simulink model "GFL_inverter"  (R2025a)
settings: Solver=ode4  StartTime=0.0  StopTime=8.5  FixedStep=1e-6  RelTol=1e-3
values from neighbouring files (symbols this model uses):
  An1 = amp1*funn    [dq_saopin_for_GFL_inverter.m]
  An2 = 0    [dq_saopin_for_GFL_inverter.m]
  An3 = 0    [dq_saopin_for_GFL_inverter.m]
  An4 = 0    [dq_saopin_for_GFL_inverter.m]
  An5 = 0    [dq_saopin_for_GFL_inverter.m]
  Ap1 = amp1*funp    [dq_saopin_for_GFL_inverter.m]
  Ap2 = 0    [dq_saopin_for_GFL_inverter.m]
  Ap3 = 0    [dq_saopin_for_GFL_inverter.m]
  Ap4 = 0    [dq_saopin_for_GFL_inverter.m]
  Ap5 = 0    [dq_saopin_for_GFL_inverter.m]
  hp1 = f    [dq_saopin_for_GFL_inverter.m]
  hp2 = f    [dq_saopin_for_GFL_inverter.m]
  hp3 = f    [dq_saopin_for_GFL_inverter.m]
  hp4 = f    [dq_saopin_for_GFL_inverter.m]
  hp5 = f    [dq_saopin_for_GFL_inverter.m]
  t_inj = 7.5    [dq_saopin_for_GFL_inverter.m]
  Ts = 5e-6    (= 5e-06)    [dq_saopin_for_GFL_inverter.m]
undefined symbols (not defined in the file or in its folder): DiscIntNeverNeededParam, level
libraries: powerlib_extras x37, spsControlledVoltageSourceLib x18, spsThreePhaseVIMeasurementLib x7, slpidlib x4, simulink_extras x4, spsabctodq0Lib x3, spsSeriesRLCBranchLib x2, spsUniversalBridgeLib x2, spsMultimeterLib x2, spsThreePhaseProgrammableVoltageSourceLib x1, spsGroundLib x1, spsIGBTDiodeLib x1
(part 2 of 2)

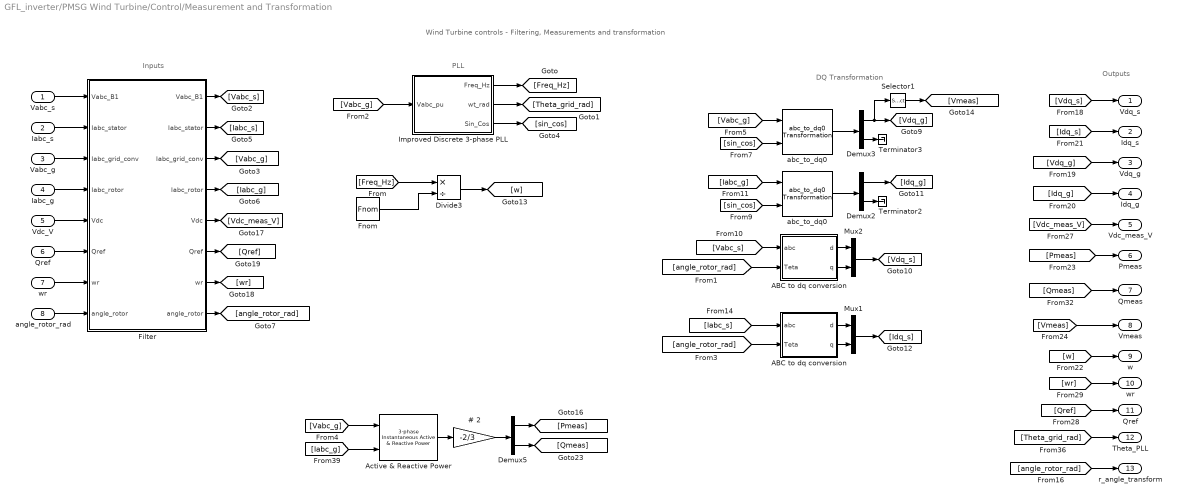
== system GFL_inverter/PMSG Wind Turbine/Control/Measurement and Transformation ==
  note: Wind Turbine controls - Filtering, Measurements and transformation
  note: Outputs
  note: Inputs
  note: PLL
  note: DQ Transformation
  Vabc_s : Inport
  Iabc_s : Inport  Port=2
  Vabc_g : Inport  Port=3
  Iabc_g : Inport  Port=4
  Vdc_V : Inport  Port=5
  Qref : Inport  Port=6
  wr : Inport  Port=7
  angle_rotor_rad : Inport  Port=8
  " Improved Discrete 3-phase PLL" : Subsystem  AncestorBlock=|  mask(Discrete 3-phase PLL){Fmin=0.75*Fnom, Par_Init=[0 Fnom], ParK=[5 3.2 1 50], Ts=Ts}
      | powerlib_extras/Discrete 
      | Control Blocks/Discrete
      | 3-phase PLL
      mask prompts: Fmin "Minimum frequency (Hz):"; Par_Init "Initial inputs:[ Phase(degrees)   Frequency(Hz) ]"; ParK "Regulator gains [ Kp1 Kp2  Ki1  Ki2 ]"; Ts "Sample time:"
      mask help:
      | This Phase Locked Loop (PLL) system can be used  to synchronize on a set of variable frequency, three-phase sinusoidal signals.
      |
      | Input 1: Vector containing the normalized
      |              three-phase signals [Va Vb Vc]
      | Output 1:  Measured frequency (Hz) = w/(2pi)
      | Output 2:  Ramp w.t   varying between  0 and 2*pi,
      | synchronized on zero crossings of the fundamental (positive-sequence) of phase A.
      | Output 3: Vector [sin(wt) cos(wt)]
      mask init:
      | Kp1=ParK(1);
      | Kp2=ParK(2);
      | Ki1=ParK(3);
      | Ki2=ParK(4);
      | Phase_Init=Par_Init(1);
      | Finit=Par_Init(2);
      | power_initmask();
      settings: OpenFcn=power_openblockproxy();
  # 2 : Gain  Gain=-2/3  SaturateOnIntegerOverflow=on  OutDataTypeStr=Inherit: Same as input  ParamDataTypeStr=Inherit: Same as input
  "ABC to dq conversion " : Subsystem
  ABC to dq conversion : Subsystem
  Active & Reactive Power : powerlib_extras/Measurements/3-phase  Instantaneous  Active & Reactive Power
  Demux2 : Demux  Outputs=[2 1]
      settings: DisplayOption=none
  Demux3 : Demux  Outputs=[2 1]
      settings: DisplayOption=none
  Demux5 : Demux  Outputs=2
      settings: DisplayOption=none
  Divide3 : Product  Inputs=*/
  Filter : Subsystem  mask{Freq=1e4, Zeta1=0.707, Ts=Ts}
      mask prompts: Freq "Cut-off frequency (Hz):"; Zeta1 "Damping factor Zeta:"; Ts "Sample time"
  Fnom : Constant  Value=Fnom
  Mux1 : Mux  Inputs=2
  Mux2 : Mux  Inputs=2
  Selector1 : Selector  InputPortWidth=2  IndexOptions=Index vector (dialog)  Indices=1  OutputSizes=[(-2)]
  Terminator2 : Terminator
  Terminator3 : Terminator
  abc_to_dq0 : powerlib_extras/Measurements/abc_to_dq0 Transformation
  "abc_to_dq0 " : powerlib_extras/Measurements/abc_to_dq0 Transformation
  Vdq_s : Outport
  Idq_s : Outport  Port=2
  Vdq_g : Outport  Port=3
  Idq_g : Outport  Port=4
  Vdc_meas_V : Outport  Port=5
  Pmeas : Outport  Port=6
  Qmeas : Outport  Port=7
  Vmeas : Outport  Port=8
  w : Outport  Port=9
  "wr " : Outport  Port=10
  "Qref " : Outport  Port=11
  Theta_PLL : Outport  Port=12
  r_angle_transform : Outport  Port=13
  wires:
  angle_rotor_rad/1 -> Filter/8(angle_rotor)
  Filter/8("angle_rotor ") -> [angle_rotor_rad]
  Filter/7("wr ") -> [wr]
  Filter/6("Qref ") -> [Qref]
  Filter/5("Vdc ") -> [Vdc_meas_V]
  Filter/4("Iabc_rotor ") -> [Iabc_g]
  Filter/3("Iabc_grid_conv ") -> [Vabc_g]
  Filter/2("Iabc_stator ") -> [Iabc_s]
  Filter/1("Vabc_B1 ") -> [Vabc_s]
  [wr] -> "wr "/1
  [Qref] -> "Qref "/1
  [Vdc_meas_V] -> Vdc_meas_V/1
  wr/1 -> Filter/7(wr)
  Qref/1 -> Filter/6(Qref)
  Vdc_V/1 -> Filter/5(Vdc)
  Iabc_g/1 -> Filter/4(Iabc_rotor)
  Vabc_g/1 -> Filter/3(Iabc_grid_conv)
  Iabc_s/1 -> Filter/2(Iabc_stator)
  Vabc_s/1 -> Filter/1(Vabc_B1)
  [angle_rotor_rad] -> "ABC to dq conversion "/2(Teta)
  [Vmeas] -> Vmeas/1
  [Pmeas] -> Pmeas/1
  [w] -> w/1
  [Idq_s] -> Idq_s/1
  [Idq_g] -> Idq_g/1
  [Vdq_g] -> Vdq_g/1
  [Vdq_s] -> Vdq_s/1
  Demux2/1 -> [Idq_g]
  [Iabc_s] -> "ABC to dq conversion "/1(abc)
  [Iabc_g] -> "abc_to_dq0 "/1
  [Vabc_s] -> ABC to dq conversion/1(abc)
  [sin_cos] -> "abc_to_dq0 "/2
  [sin_cos] -> abc_to_dq0/2
  [Vabc_g] -> abc_to_dq0/1
  [Freq_Hz] -> Divide3/1
  Divide3/1 -> [w]
  Fnom/1 -> Divide3/2
  "abc_to_dq0 "/1 -> Demux2/1
  Demux2/2 -> Terminator2/1
  abc_to_dq0/1 -> Demux3/1
  Demux3/2 -> Terminator3/1
  Demux3/1 -> [Vdq_g], Selector1/1
  [Qmeas] -> Qmeas/1
  [Theta_grid_rad] -> Theta_PLL/1
  [angle_rotor_rad] -> r_angle_transform/1
  [Vabc_g] -> " Improved Discrete 3-phase PLL"/1(Vabc_pu)
  " Improved Discrete 3-phase PLL"/2(wt_rad) -> [Theta_grid_rad]
  " Improved Discrete 3-phase PLL"/3(Sin_Cos) -> [sin_cos]
  " Improved Discrete 3-phase PLL"/1(Freq_Hz) -> [Freq_Hz]
  [Vabc_g] -> Active & Reactive Power/1
  [Iabc_g] -> Active & Reactive Power/2
  Demux5/1 -> [Pmeas]
  Demux5/2 -> [Qmeas]
  Active & Reactive Power/1 -> # 2/1
  # 2/1 -> Demux5/1
  Selector1/1 -> [Vmeas]
  [angle_rotor_rad] -> ABC to dq conversion/2(Teta)
  ABC to dq conversion/1(d) -> Mux2/1
  ABC to dq conversion/2(q) -> Mux2/2
  Mux2/1 -> [Vdq_s]
  "ABC to dq conversion "/1(d) -> Mux1/1
  "ABC to dq conversion "/2(q) -> Mux1/2
  Mux1/1 -> [Idq_s]

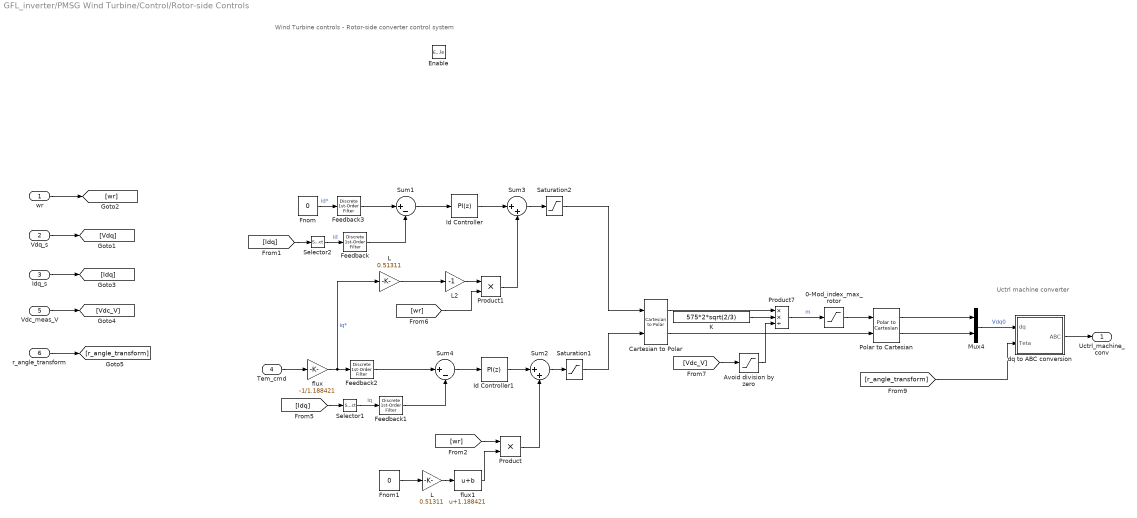
== system GFL_inverter/PMSG Wind Turbine/Control/Rotor-side Controls ==
  note: Wind Turbine controls - Rotor-side converter control system
  note: Uctrl machine converter
  wr : Inport
  " Vdq_s" : Inport  Port=2
  Idq_s : Inport  Port=3
  Tem_cmd : Inport  Port=4
  Vdc_meas_V : Inport  Port=5
  r_angle_transform : Inport  Port=6
  Enable : EnablePort
  0-Mod_index_max_rotor : Saturate  UpperLimit=2  LowerLimit=0
  Avoid division by zero : Saturate  UpperLimit=inf  LowerLimit=1e-6
  Cartesian to Polar : simulink_extras/Transformations/Cartesian to Polar
  Feedback{,1..3} (4 alike) : powerlib_extras/Discrete  Control Blocks/Discrete 1st-Order Filter  FilterType=Lowpass  Tc=Fb_time_const  Ts=Ts  Initialize=on  Vac_Init=[0 -25 60]  Vdc_Init=0  PlotResponse=off  param1=[1 500 0.1]
  Fnom : Constant  Value=0
  Fnom1 : Constant  Value=0
  Id Controller : slpidlib/PID Controller  Controller=PI  Form=Parallel  TimeDomain=Discrete-time  UseExternalTs=off  SampleTime=Ts  IntegratorMethod=Forward Euler  FilterMethod=Forward Euler  ControllerParametersSource=internal  P=0.03*2129.991/469.486  I=(0.03/0.05)*2129.991/469.486  UseKiTs=off  D=0  UseExternalDerivativeSource=off  N=100  UseFilter=on  TunerSelectOption=Transfer Function Based (PID Tuner App)  ZeroCross=off  InitialConditionSource=internal  InitialConditionForIntegrator=0  InitialConditionForFilter=0  DifferentiatorICPrevScaledInput=0  ExternalReset=none  TrackingMode=off  Kt=1  LimitOutput=off  SatLimitsSource=internal  UpperSaturationLimit=2  LowerSaturationLimit=-2  LinearizeAsGain=off  AntiWindupMode=clamping  Kb=1  LimitIntegrator=off  UpperIntegratorSaturationLimit=inf  LowerIntegratorSaturationLimit=-inf  POutMin=[]  POutMax=[]  IOutMin=[]  IOutMax=[]  DOutMin=[]  DOutMax=[]  NOutMin=[]  NOutMax=[]  SumOutMin=[]  SumOutMax=[]  SaturationOutMin=[]  SaturationOutMax=[]  PParamMin=[]  PParamMax=[]  IParamMin=[]  IParamMax=[]  DParamMin=[]  DParamMax=[]  NParamMin=[]  NParamMax=[]  KbParamMin=[]  KbParamMax=[]  KtParamMin=[]  KtParamMax=[]  KbOutMin=[]  KbOutMax=[]  KtOutMin=[]  KtOutMax=[]  IntegratorOutMin=[]  IntegratorOutMax=[]  FilterOutMin=[]  FilterOutMax=[]  SumI1OutMin=[]  SumI1OutMax=[]  SumI2OutMin=[]  SumI2OutMax=[]  SumI3OutMin=[]  SumI3OutMax=[]  SumI4OutMin=[]  SumI4OutMax=[]  SumDOutMin=[]  SumDOutMax=[]  DifferentiatorOutMin=[]  DifferentiatorOutMax=[]  FilterDiffOutCoefMin=[]  FilterDiffOutCoefMax=[]  ReciprocalOutMin=[]  ReciprocalOutMax=[]  SumDenOutMin=[]  SumDenOutMax=[]  SumNumOutMin=[]  SumNumOutMax=[]  DivideOutMin=[]  DivideOutMax=[]  UdiffTsProdOutMin=[]  UdiffTsProdOutMax=[]  NTsProdOutMin=[]  NTsProdOutMax=[]  UintegralTsProdOutMin=[]  UintegralTsProdOutMax=[]  UngainTsProdOutMin=[]  UngainTsProdOutMax=[]  ClampingZeroOutDataTypeStr=Inherit: Inherit via back propagation  ClampingZeroOutMin=[]  ClampingZeroOutMax=[]  FilterDenConstantOutDataTypeStr=Inherit: Inherit via back propagation  FilterDenConstantOutMin=[]  FilterDenConstantOutMax=[]  PCopyOutDataTypeStr=Inherit: Inherit via back propagation  PCopyOutMin=[]  PCopyOutMax=[]  NCopyOutDataTypeStr=Inherit: Inherit via back propagation  NCopyOutMin=[]  NCopyOutMax=[]  IntegratorContinuousStateAttributes=''  IntegratorStateMustResolveToSignalObject=off  IntegratorRTWStateStorageClass=Auto  FilterContinuousStateAttributes=''  FilterStateMustResolveToSignalObject=off  FilterRTWStateStorageClass=Auto  ParallelPVariant=InternalParameters  IdealPVariant=Disabled  IVariant=InternalParameters  DVariant=Disabled  IntegratorVariant=Discrete  SatVariant=Disabled  AWVariant=Passthrough  PCopyVariant=Disabled  TRVariant=Disabled  FdbkBlocksVariant=Forward  IdealPFdbkVariant=Disabled  SatFdbkVariant=Disabled  DerivativeFilterVariant=Disabled  NVariant=Disabled  NCopyVariant=Disabled_SignalSpec  FilterICVariant=Disabled  IntegratorICVariant=InternalICs  ExternalResetVariant=Disabled  TRSumVariant=Passthrough  SumFdbkVariant=Disabled  SumVariant=Sum_PI  TsampFilterVariant=InternalTs  TsampNgainVariant=Passthrough  TsampIntegralVariant=Disabled_SignalSpec  ExternalSaturationOutDataTypeStr=Inherit: Same as second input  DerivativeSourceVariant=Disabled  PreIntVariant=InternalPreInt
  Id Controller1 : slpidlib/PID Controller  Controller=PI  Form=Parallel  TimeDomain=Discrete-time  UseExternalTs=off  SampleTime=Ts  IntegratorMethod=Forward Euler  FilterMethod=Forward Euler  ControllerParametersSource=internal  P=0.03*2129.991/469.486  I=(0.03/0.05)*2129.991/469.486  UseKiTs=off  D=0  UseExternalDerivativeSource=off  N=100  UseFilter=on  TunerSelectOption=Transfer Function Based (PID Tuner App)  ZeroCross=off  InitialConditionSource=internal  InitialConditionForIntegrator=0  InitialConditionForFilter=0  DifferentiatorICPrevScaledInput=0  ExternalReset=none  TrackingMode=off  Kt=1  LimitOutput=off  SatLimitsSource=internal  UpperSaturationLimit=2  LowerSaturationLimit=-2  LinearizeAsGain=off  AntiWindupMode=clamping  Kb=1  LimitIntegrator=off  UpperIntegratorSaturationLimit=inf  LowerIntegratorSaturationLimit=-inf  POutMin=[]  POutMax=[]  IOutMin=[]  IOutMax=[]  DOutMin=[]  DOutMax=[]  NOutMin=[]  NOutMax=[]  SumOutMin=[]  SumOutMax=[]  SaturationOutMin=[]  SaturationOutMax=[]  PParamMin=[]  PParamMax=[]  IParamMin=[]  IParamMax=[]  DParamMin=[]  DParamMax=[]  NParamMin=[]  NParamMax=[]  KbParamMin=[]  KbParamMax=[]  KtParamMin=[]  KtParamMax=[]  KbOutMin=[]  KbOutMax=[]  KtOutMin=[]  KtOutMax=[]  IntegratorOutMin=[]  IntegratorOutMax=[]  FilterOutMin=[]  FilterOutMax=[]  SumI1OutMin=[]  SumI1OutMax=[]  SumI2OutMin=[]  SumI2OutMax=[]  SumI3OutMin=[]  SumI3OutMax=[]  SumI4OutMin=[]  SumI4OutMax=[]  SumDOutMin=[]  SumDOutMax=[]  DifferentiatorOutMin=[]  DifferentiatorOutMax=[]  FilterDiffOutCoefMin=[]  FilterDiffOutCoefMax=[]  ReciprocalOutMin=[]  ReciprocalOutMax=[]  SumDenOutMin=[]  SumDenOutMax=[]  SumNumOutMin=[]  SumNumOutMax=[]  DivideOutMin=[]  DivideOutMax=[]  UdiffTsProdOutMin=[]  UdiffTsProdOutMax=[]  NTsProdOutMin=[]  NTsProdOutMax=[]  UintegralTsProdOutMin=[]  UintegralTsProdOutMax=[]  UngainTsProdOutMin=[]  UngainTsProdOutMax=[]  ClampingZeroOutDataTypeStr=Inherit: Inherit via back propagation  ClampingZeroOutMin=[]  ClampingZeroOutMax=[]  FilterDenConstantOutDataTypeStr=Inherit: Inherit via back propagation  FilterDenConstantOutMin=[]  FilterDenConstantOutMax=[]  PCopyOutDataTypeStr=Inherit: Inherit via back propagation  PCopyOutMin=[]  PCopyOutMax=[]  NCopyOutDataTypeStr=Inherit: Inherit via back propagation  NCopyOutMin=[]  NCopyOutMax=[]  IntegratorContinuousStateAttributes=''  IntegratorStateMustResolveToSignalObject=off  IntegratorRTWStateStorageClass=Auto  FilterContinuousStateAttributes=''  FilterStateMustResolveToSignalObject=off  FilterRTWStateStorageClass=Auto  ParallelPVariant=InternalParameters  IdealPVariant=Disabled  IVariant=InternalParameters  DVariant=Disabled  IntegratorVariant=Discrete  SatVariant=Disabled  AWVariant=Passthrough  PCopyVariant=Disabled  TRVariant=Disabled  FdbkBlocksVariant=Forward  IdealPFdbkVariant=Disabled  SatFdbkVariant=Disabled  DerivativeFilterVariant=Disabled  NVariant=Disabled  NCopyVariant=Disabled_SignalSpec  FilterICVariant=Disabled  IntegratorICVariant=InternalICs  ExternalResetVariant=Disabled  TRSumVariant=Passthrough  SumFdbkVariant=Disabled  SumVariant=Sum_PI  TsampFilterVariant=InternalTs  TsampNgainVariant=Passthrough  TsampIntegralVariant=Disabled_SignalSpec  ExternalSaturationOutDataTypeStr=Inherit: Same as second input  DerivativeSourceVariant=Disabled  PreIntVariant=InternalPreInt
  K : Constant  Value=575*2*sqrt(2/3)
  L : Gain  Gain=0.51311
  "L  " : Gain  Gain=0.51311
  L2 : Gain  Gain=-1
  Mux4 : Mux  Inputs=2
  Polar to Cartesian : simulink_extras/Transformations/Polar to Cartesian
  Product : Product  RndMeth=Zero
  Product1 : Product  RndMeth=Zero
  Product7 : Product  Inputs=**/  InputSameDT=on  SaturateOnIntegerOverflow=on  OutDataTypeStr=Inherit: Same as first input
  Saturation1 : Saturate  UpperLimit=inf  LowerLimit=-inf  SampleTime=Ts
  Saturation2 : Saturate  UpperLimit=inf  LowerLimit=-inf  SampleTime=Ts
  Selector1 : Selector  InputPortWidth=2  IndexOptions=Index vector (dialog)  Indices=2  OutputSizes=[(-2)]
  Selector2 : Selector  InputPortWidth=2  IndexOptions=Index vector (dialog)  Indices=1  OutputSizes=[(-2)]
  Sum1 : Sum  Inputs=|+-  InputSameDT=on  SaturateOnIntegerOverflow=on  OutDataTypeStr=Inherit: Same as first input
  Sum2 : Sum  Inputs=|++  InputSameDT=on  SaturateOnIntegerOverflow=on  OutDataTypeStr=Inherit: Same as first input
  Sum3 : Sum  Inputs=|++  InputSameDT=on  SaturateOnIntegerOverflow=on  OutDataTypeStr=Inherit: Same as first input
  Sum4 : Sum  Inputs=|+-  InputSameDT=on  SaturateOnIntegerOverflow=on  OutDataTypeStr=Inherit: Same as first input
  "dq to ABC conversion " : Subsystem
  flux : Gain  Gain=-1/1.188421
  flux1 : Bias  Bias=1.188421  SaturateOnIntegerOverflow=off
  Uctrl_machine_conv : Outport
  wires:
  Tem_cmd/1 -> flux/1
  wr/1 -> [wr]
  " Vdq_s"/1 -> [Vdq]
  Idq_s/1 -> [Idq]
  Vdc_meas_V/1 -> [Vdc_V]
  r_angle_transform/1 -> [r_angle_transform]
  [Idq] -> Selector1/1
  Sum4/1 -> Id Controller1/1
  [Idq] -> Selector2/1
  Sum1/1 -> Id Controller/1
  Id Controller1/1 -> Sum2/1
  Id Controller/1 -> Sum3/1
  [wr] -> Product/1
  flux1/1 -> Product/2
  L/1 -> flux1/1
  "L  "/1 -> L2/1
  L2/1 -> Product1/1
  [wr] -> Product1/2
  Cartesian to Polar/1 -> Product7/1
  K/1 -> Product7/2
  Mux4/1 -> "dq to ABC conversion "/1(dq)  "Vdq0"
  Avoid division by zero/1 -> Product7/3
  [Vdc_V] -> Avoid division by zero/1
  Product7/1 -> 0-Mod_index_max_rotor/1  "m"
  Cartesian to Polar/2 -> Polar to Cartesian/2
  0-Mod_index_max_rotor/1 -> Polar to Cartesian/1
  Polar to Cartesian/1 -> Mux4/1
  Polar to Cartesian/2 -> Mux4/2
  Selector2/1 -> Feedback/1  "id"
  Feedback/1 -> Sum1/2
  Feedback1/1 -> Sum4/2
  Product1/1 -> Sum3/2
  Product/1 -> Sum2/2
  Selector1/1 -> Feedback1/1  "iq"
  [r_angle_transform] -> "dq to ABC conversion "/2(Teta)
  "dq to ABC conversion "/1(ABC) -> Uctrl_machine_conv/1
  Sum3/1 -> Saturation2/1
  Saturation2/1 -> Cartesian to Polar/1
  Sum2/1 -> Saturation1/1
  Saturation1/1 -> Cartesian to Polar/2
  flux/1 -> Feedback2/1, "L  "/1  "iq*"
  Feedback2/1 -> Sum4/1
  Feedback3/1 -> Sum1/1
  Fnom/1 -> Feedback3/1  "id*"
  Fnom1/1 -> L/1

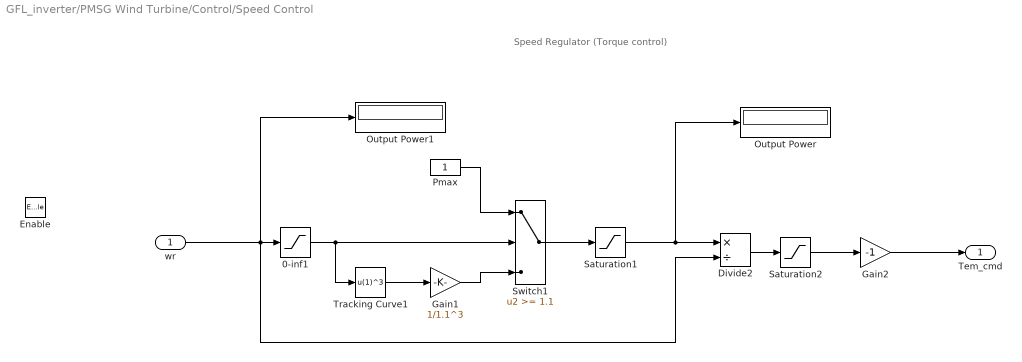
== system GFL_inverter/PMSG Wind Turbine/Control/Speed Control ==
  note: Speed Regulator
      | (Torque control)
  wr : Inport
  Enable : EnablePort
  0-inf1 : Saturate  UpperLimit=1.2  LowerLimit=0.6
  Divide2 : Product  Inputs=*/  SampleTime=Ts
  Gain1 : Gain  Gain=1/1.1^3  SampleTime=Ts
  Gain2 : Gain  Gain=-1  SampleTime=Ts
  Output Power : Display
      settings: Decimation=1000
  Output Power1 : Display
      settings: Decimation=1000
  Pmax : Constant
  Saturation1 : Saturate  UpperLimit=1  LowerLimit=-1
  Saturation2 : Saturate  UpperLimit=1.1  LowerLimit=-1.1
  Switch1 : Switch  Threshold=1.1  SaturateOnIntegerOverflow=off  InputSameDT=off
  Tracking Curve1 : Fcn  Expr=u(1)^3
  Tem_cmd : Outport
  wires:
  wr/1 -> 0-inf1/1, Divide2/2, Output Power1/1
  Pmax/1 -> Switch1/1
  0-inf1/1 -> Switch1/2, Tracking Curve1/1
  Switch1/1 -> Saturation1/1
  Divide2/1 -> Saturation2/1
  Saturation1/1 -> Divide2/1, Output Power/1
  Tracking Curve1/1 -> Gain1/1
  Gain1/1 -> Switch1/3
  Saturation2/1 -> Gain2/1
  Gain2/1 -> Tem_cmd/1

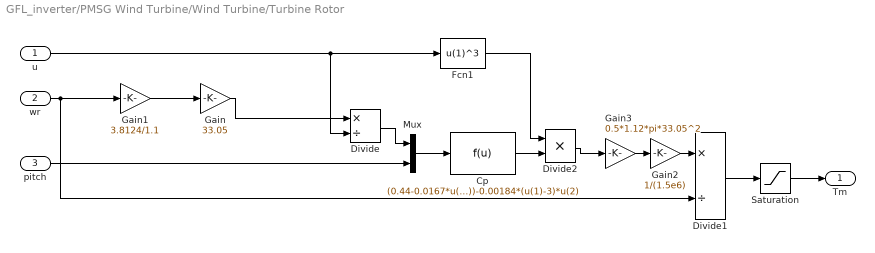
== system GFL_inverter/PMSG Wind Turbine/Wind Turbine/Turbine Rotor ==
  u : Inport
  wr : Inport  Port=2
  pitch : Inport  Port=3
  Cp : Fcn  Expr=(0.44-0.0167*u(2))*sin(pi*(u(1)-3)/15-0.3*u(2))-0.00184*(u(1)-3)*u(2)  SampleTime=Ts
  Divide : Product  Inputs=*/  SampleTime=Ts
  Divide1 : Product  Inputs=*/  SampleTime=Ts
  Divide2 : Product  Inputs=**  SampleTime=Ts
  Fcn1 : Fcn  Expr=u(1)^3  SampleTime=Ts
  Gain : Gain  Gain=33.05  SampleTime=Ts
  Gain1 : Gain  Gain=3.8124/1.1  SampleTime=Ts
  Gain2 : Gain  Gain=1/(1.5e6)  SampleTime=Ts
  Gain3 : Gain  Gain=0.5*1.12*pi*33.05^2  SampleTime=Ts
  Mux : Mux  Inputs=2
  Saturation : Saturate  UpperLimit=inf  LowerLimit=1e-2
  Tm : Outport
  wires:
  Gain/1 -> Divide/1
  u/1 -> Divide/2, Fcn1/1
  Divide/1 -> Mux/1
  Mux/1 -> Cp/1
  wr/1 -> Gain1/1, Divide1/2
  Gain1/1 -> Gain/1
  Gain2/1 -> Divide1/1
  Gain3/1 -> Gain2/1
  Divide2/1 -> Gain3/1
  Cp/1 -> Divide2/2
  Fcn1/1 -> Divide2/1
  pitch/1 -> Mux/2
  Divide1/1 -> Saturation/1
  Saturation/1 -> Tm/1

== system GFL_inverter/PMSG Wind Turbine/Wind Turbine/pitch angle controller ==
  wg : Inport
  Ref : Inport  Port=2
  "0-pitch_max " : Saturate  UpperLimit=27  LowerLimit=0  SampleTime=Ts
  Discrete PID Controller : slpidlib/PID Controller  Controller=P  Form=Parallel  TimeDomain=Discrete-time  UseExternalTs=off  SampleTime=Ts  IntegratorMethod=Forward Euler  FilterMethod=Forward Euler  ControllerParametersSource=internal  P=200  I=0  UseKiTs=off  D=0  UseExternalDerivativeSource=off  N=100  UseFilter=on  TunerSelectOption=Transfer Function Based (PID Tuner App)  ZeroCross=off  InitialConditionSource=internal  InitialConditionForIntegrator=0  InitialConditionForFilter=0  DifferentiatorICPrevScaledInput=0  ExternalReset=none  TrackingMode=off  Kt=1  LimitOutput=on  SatLimitsSource=internal  UpperSaturationLimit=27  LowerSaturationLimit=0  LinearizeAsGain=off  AntiWindupMode=clamping  Kb=1  LimitIntegrator=off  UpperIntegratorSaturationLimit=inf  LowerIntegratorSaturationLimit=-inf  POutMin=[]  POutMax=[]  IOutMin=[]  IOutMax=[]  DOutMin=[]  DOutMax=[]  NOutMin=[]  NOutMax=[]  SumOutMin=[]  SumOutMax=[]  SaturationOutMin=[]  SaturationOutMax=[]  PParamMin=[]  PParamMax=[]  IParamMin=[]  IParamMax=[]  DParamMin=[]  DParamMax=[]  NParamMin=[]  NParamMax=[]  KbParamMin=[]  KbParamMax=[]  KtParamMin=[]  KtParamMax=[]  KbOutMin=[]  KbOutMax=[]  KtOutMin=[]  KtOutMax=[]  IntegratorOutMin=[]  IntegratorOutMax=[]  FilterOutMin=[]  FilterOutMax=[]  SumI1OutMin=[]  SumI1OutMax=[]  SumI2OutMin=[]  SumI2OutMax=[]  SumI3OutMin=[]  SumI3OutMax=[]  SumI4OutMin=[]  SumI4OutMax=[]  SumDOutMin=[]  SumDOutMax=[]  DifferentiatorOutMin=[]  DifferentiatorOutMax=[]  FilterDiffOutCoefMin=[]  FilterDiffOutCoefMax=[]  ReciprocalOutMin=[]  ReciprocalOutMax=[]  SumDenOutMin=[]  SumDenOutMax=[]  SumNumOutMin=[]  SumNumOutMax=[]  DivideOutMin=[]  DivideOutMax=[]  UdiffTsProdOutMin=[]  UdiffTsProdOutMax=[]  NTsProdOutMin=[]  NTsProdOutMax=[]  UintegralTsProdOutMin=[]  UintegralTsProdOutMax=[]  UngainTsProdOutMin=[]  UngainTsProdOutMax=[]  ClampingZeroOutDataTypeStr=Inherit: Inherit via back propagation  ClampingZeroOutMin=[]  ClampingZeroOutMax=[]  FilterDenConstantOutDataTypeStr=Inherit: Inherit via back propagation  FilterDenConstantOutMin=[]  FilterDenConstantOutMax=[]  PCopyOutDataTypeStr=Inherit: Inherit via back propagation  PCopyOutMin=[]  PCopyOutMax=[]  NCopyOutDataTypeStr=Inherit: Inherit via back propagation  NCopyOutMin=[]  NCopyOutMax=[]  IntegratorContinuousStateAttributes=''  IntegratorStateMustResolveToSignalObject=off  IntegratorRTWStateStorageClass=Auto  FilterContinuousStateAttributes=''  FilterStateMustResolveToSignalObject=off  FilterRTWStateStorageClass=Auto  ParallelPVariant=InternalParameters  IdealPVariant=Disabled  IVariant=Disabled  DVariant=Disabled  IntegratorVariant=Disabled  SatVariant=Enabled  AWVariant=Disabled  PCopyVariant=Disabled  TRVariant=Disabled  FdbkBlocksVariant=Forward  IdealPFdbkVariant=Disabled  SatFdbkVariant=Disabled  DerivativeFilterVariant=Disabled  NVariant=Disabled  NCopyVariant=Disabled_SignalSpec  FilterICVariant=Disabled  IntegratorICVariant=Disabled  ExternalResetVariant=Disabled  TRSumVariant=Passthrough  SumFdbkVariant=Disabled  SumVariant=Passthrough_P  TsampFilterVariant=InternalTs  TsampNgainVariant=Passthrough  TsampIntegralVariant=Disabled_SignalSpec  ExternalSaturationOutDataTypeStr=Inherit: Same as second input  DerivativeSourceVariant=Disabled  PreIntVariant=InternalPreInt
  Rate Limiter : RateLimiter  RisingSlewLimit=10  FallingSlewLimit=-10
  Sum3 : Sum  Inputs=|+-  SampleTime=Ts
  t=Pitch_time_constant1 : powerlib_extras/Discrete  Control Blocks/Discrete 1st-Order Filter  FilterType=Lowpass  Tc=0.02  Ts=Ts  Initialize=on  Vac_Init=[0.8 -25 60]*0  Vdc_Init=0  PlotResponse=off  param1=[1 500 0.1]
  pitch : Outport
  wires:
  Sum3/1 -> Discrete PID Controller/1
  wg/1 -> Sum3/1
  Ref/1 -> Sum3/2
  Rate Limiter/1 -> "0-pitch_max "/1
  "0-pitch_max "/1 -> t=Pitch_time_constant1/1
  t=Pitch_time_constant1/1 -> pitch/1
  Discrete PID Controller/1 -> Rate Limiter/1

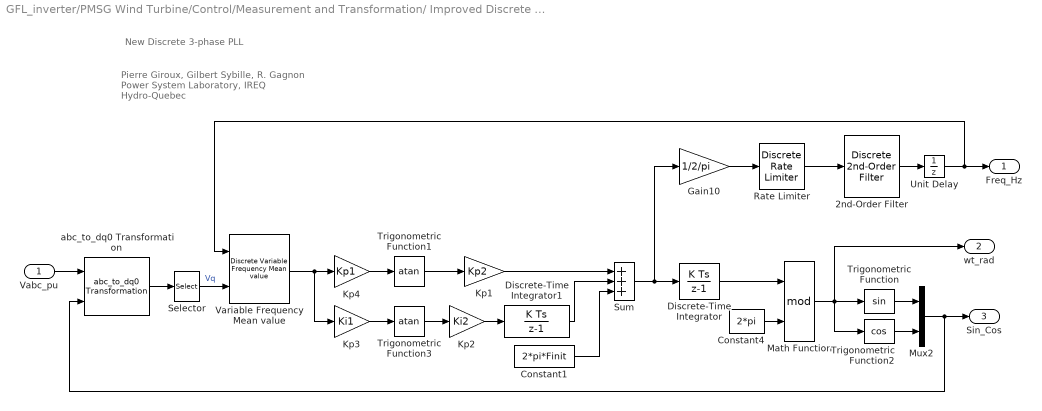
== system GFL_inverter/PMSG Wind Turbine/Control/Measurement and Transformation/ Improved Discrete 3-phase PLL ==
  note: New Discrete 3-phase PLL
  note: Pierre Giroux, Gilbert Sybille, R. Gagnon
      | Power System Laboratory, IREQ
      | Hydro-Quebec
  Vabc_pu : Inport  PortDimensions=3
  2nd-Order Filter : powerlib_extras/Discrete  Control Blocks/Discrete  2nd-Order Filter  FilterType=Lowpass  Fo=25  Zeta=0.707  Ts=Ts  Initialize=on  Vac_Init=[0 0 Finit]  Vdc_Init=Finit  PlotResponse=off  param1=[1 500 0.1]
  Constant1 : Constant  Value=2*pi*Finit
  Constant4 : Constant  Value=2*pi
  Discrete-Time Integrator : DiscreteIntegrator  SampleTime=Ts  ICPrevOutput=DiscIntNeverNeededParam  ICPrevScaledInput=DiscIntNeverNeededParam
  Discrete-Time Integrator1 : DiscreteIntegrator  gainval=1  SampleTime=Ts  LimitOutput=on  UpperSaturationLimit=2*pi*5  LowerSaturationLimit=-2*pi*5  ICPrevOutput=DiscIntNeverNeededParam  ICPrevScaledInput=DiscIntNeverNeededParam
  Gain10 : Gain  Gain=1/2/pi  SaturateOnIntegerOverflow=on  OutDataTypeStr=Inherit: Same as input  ParamDataTypeStr=Inherit: Same as input
  Kp1 : Gain  Gain=Kp2  SaturateOnIntegerOverflow=on  OutDataTypeStr=Inherit: Same as input  ParamDataTypeStr=Inherit: Same as input
  Kp2 : Gain  Gain=Ki2  SaturateOnIntegerOverflow=on  OutDataTypeStr=Inherit: Same as input  ParamDataTypeStr=Inherit: Same as input
  Kp3 : Gain  Gain=Ki1  SaturateOnIntegerOverflow=on  OutDataTypeStr=Inherit: Same as input  ParamDataTypeStr=Inherit: Same as input
  Kp4 : Gain  Gain=Kp1  SaturateOnIntegerOverflow=on  OutDataTypeStr=Inherit: Same as input  ParamDataTypeStr=Inherit: Same as input
  Math Function : Math  Operator=mod  SignedPower=on
  Mux2 : Mux  Inputs=2
  Rate Limiter : powerlib_extras/Discrete  Control Blocks/Discrete Rate Limiter  R=12  F=-12  Vinit=Finit  Ts=Ts
  Selector : Selector  InputPortWidth=3  IndexOptions=Index vector (dialog)  Indices=2  OutputSizes=1
  Sum : Sum  Inputs=+++
  Trigonometric Function : Trigonometry
  Trigonometric Function1 : Trigonometry  Operator=atan
  Trigonometric Function2 : Trigonometry  Operator=cos
  Trigonometric Function3 : Trigonometry  Operator=atan
  Unit Delay : UnitDelay  InitialCondition=Finit  SampleTime=Ts
  Variable Frequency Mean value : powerlib_extras/Discrete Measurements/Discrete Variable Frequency Mean value  Finit=Finit  Fmin=Fmin  Vinit=0  Ts=Ts
  abc_to_dq0 Transformation : powerlib_extras/Measurements/abc_to_dq0 Transformation
  Freq_Hz : Outport
  wt_rad : Outport  Port=2
  Sin_Cos : Outport  Port=3
  wires:
  Vabc_pu/1 -> abc_to_dq0 Transformation/1
  abc_to_dq0 Transformation/1 -> Selector/1
  Constant4/1 -> Math Function/2
  Math Function/1 -> Trigonometric Function/1, Trigonometric Function2/1, wt_rad/1
  Trigonometric Function/1 -> Mux2/1
  Trigonometric Function2/1 -> Mux2/2
  Mux2/1 -> Sin_Cos/1, abc_to_dq0 Transformation/2
  Gain10/1 -> Rate Limiter/1
  Rate Limiter/1 -> 2nd-Order Filter/1
  2nd-Order Filter/1 -> Unit Delay/1
  Selector/1 -> Variable Frequency Mean value/2  "Vq"
  Kp4/1 -> Trigonometric Function1/1
  Trigonometric Function1/1 -> Kp1/1
  Constant1/1 -> Sum/3
  Variable Frequency Mean value/1 -> Kp4/1, Kp3/1
  Kp3/1 -> Trigonometric Function3/1
  Trigonometric Function3/1 -> Kp2/1
  Kp2/1 -> Discrete-Time Integrator1/1
  Sum/1 -> Discrete-Time Integrator/1, Gain10/1
  Unit Delay/1 -> Freq_Hz/1, Variable Frequency Mean value/1
  Discrete-Time Integrator/1 -> Math Function/1
  Kp1/1 -> Sum/1
  Discrete-Time Integrator1/1 -> Sum/2

== system GFL_inverter/PMSG Wind Turbine/Control/Measurement and Transformation/ABC to dq conversion  ==
  abc : Inport
  Teta : Inport  Port=2
  Fcn : Fcn  Expr=sin(u)
  Fcn1 : Fcn  Expr=cos(u)
  Gain : Gain  Gain=2/3  SaturateOnIntegerOverflow=on  OutDataTypeStr=Inherit: Same as input  ParamDataTypeStr=Inherit: Same as input
  Gain1 : Gain  Gain=2/3  SaturateOnIntegerOverflow=on  OutDataTypeStr=Inherit: Same as input  ParamDataTypeStr=Inherit: Same as input
  Mux : Mux  Inputs=[1 1 3]
  id : Fcn  Expr=u[1]*u[3]+(1.7320508*u[2]-u[1])*u[4]*0.5+(-u[1]-1.7320508*u[2])*u[5]*0.5
  iq : Fcn  Expr=-u[2]*u[3]+(u[2]+1.7320508*u[1])*u[4]*0.5+(u[2]-1.7320508*u[1])*u[5]*0.5
  d : Outport  InitialOutput=0
  q : Outport  Port=2  InitialOutput=0
  wires:
  Fcn/1 -> Mux/2
  Fcn1/1 -> Mux/1
  Teta/1 -> Fcn1/1, Fcn/1
  Mux/1 -> iq/1, id/1
  abc/1 -> Mux/3
  iq/1 -> Gain1/1
  id/1 -> Gain/1
  Gain/1 -> d/1
  Gain1/1 -> q/1

== system GFL_inverter/PMSG Wind Turbine/Control/Measurement and Transformation/ABC to dq conversion ==
  abc : Inport
  Teta : Inport  Port=2
  Fcn : Fcn  Expr=sin(u)
  Fcn1 : Fcn  Expr=cos(u)
  Gain : Gain  Gain=2/3  SaturateOnIntegerOverflow=on  OutDataTypeStr=Inherit: Same as input  ParamDataTypeStr=Inherit: Same as input
  Gain1 : Gain  Gain=2/3  SaturateOnIntegerOverflow=on  OutDataTypeStr=Inherit: Same as input  ParamDataTypeStr=Inherit: Same as input
  Mux : Mux  Inputs=[1 1 3]
  id : Fcn  Expr=u[1]*u[3]+(1.7320508*u[2]-u[1])*u[4]*0.5+(-u[1]-1.7320508*u[2])*u[5]*0.5
  iq : Fcn  Expr=-u[2]*u[3]+(u[2]+1.7320508*u[1])*u[4]*0.5+(u[2]-1.7320508*u[1])*u[5]*0.5
  d : Outport  InitialOutput=0
  q : Outport  Port=2  InitialOutput=0
  wires:
  Fcn/1 -> Mux/2
  Fcn1/1 -> Mux/1
  Teta/1 -> Fcn1/1, Fcn/1
  Mux/1 -> iq/1, id/1
  abc/1 -> Mux/3
  iq/1 -> Gain1/1
  id/1 -> Gain/1
  Gain/1 -> d/1
  Gain1/1 -> q/1

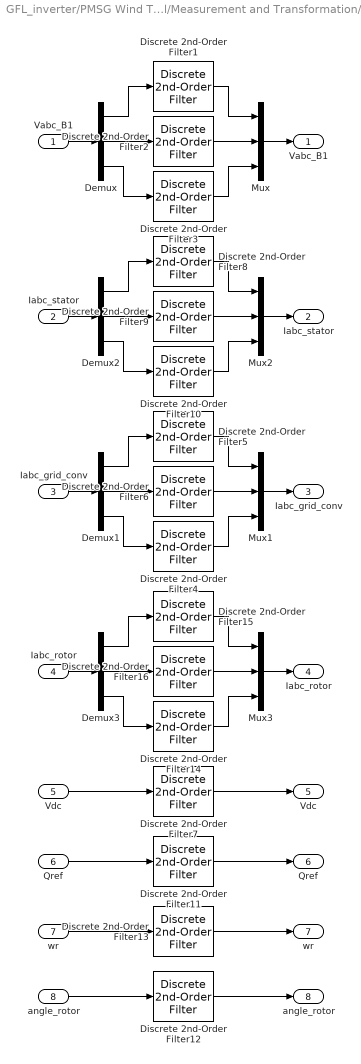
== system GFL_inverter/PMSG Wind Turbine/Control/Measurement and Transformation/Filter ==
  Vabc_B1 : Inport
  Iabc_stator : Inport  Port=2
  Iabc_grid_conv : Inport  Port=3
  Iabc_rotor : Inport  Port=4
  Vdc : Inport  Port=5
  Qref : Inport  Port=6
  wr : Inport  Port=7
  angle_rotor : Inport  Port=8
  Demux{,1..3} (4 alike) : Demux  Outputs=3
      settings: DisplayOption=none
  Discrete 2nd-Order Filter{1..6,8..16} (15 alike) : powerlib_extras/Discrete  Control Blocks/Discrete  2nd-Order Filter  FilterType=Lowpass  Fo=Freq  Zeta=Zeta1  Ts=Ts  Initialize=off  Vac_Init=[0.8 -25 60]  Vdc_Init=-0.4  PlotResponse=off  param1=[1 500 1]
  Discrete 2nd-Order Filter7 : powerlib_extras/Discrete  Control Blocks/Discrete  2nd-Order Filter  FilterType=Lowpass  Fo=Freq  Zeta=Zeta1  Ts=Ts  Initialize=on  Vac_Init=[0.8 -25 60]*0  Vdc_Init=Vdc_nom  PlotResponse=off  param1=[1 500 1]
  Mux{,1..3} (4 alike) : Mux  Inputs=3
  "Vabc_B1 " : Outport
  "Iabc_stator " : Outport  Port=2
  "Iabc_grid_conv " : Outport  Port=3
  "Iabc_rotor " : Outport  Port=4
  "Vdc " : Outport  Port=5
  "Qref " : Outport  Port=6
  "wr " : Outport  Port=7
  "angle_rotor " : Outport  Port=8
  wires:
  Discrete 2nd-Order Filter12/1 -> "angle_rotor "/1
  angle_rotor/1 -> Discrete 2nd-Order Filter12/1
  Discrete 2nd-Order Filter11/1 -> "Qref "/1
  Qref/1 -> Discrete 2nd-Order Filter11/1
  Mux3/1 -> "Iabc_rotor "/1
  Iabc_rotor/1 -> Demux3/1
  Discrete 2nd-Order Filter14/1 -> Mux3/3
  Discrete 2nd-Order Filter16/1 -> Mux3/2
  Discrete 2nd-Order Filter15/1 -> Mux3/1
  Demux3/3 -> Discrete 2nd-Order Filter14/1
  Demux3/2 -> Discrete 2nd-Order Filter16/1
  Demux3/1 -> Discrete 2nd-Order Filter15/1
  Discrete 2nd-Order Filter13/1 -> "wr "/1
  wr/1 -> Discrete 2nd-Order Filter13/1
  Mux2/1 -> "Iabc_stator "/1
  Iabc_stator/1 -> Demux2/1
  Discrete 2nd-Order Filter10/1 -> Mux2/3
  Discrete 2nd-Order Filter9/1 -> Mux2/2
  Discrete 2nd-Order Filter8/1 -> Mux2/1
  Demux2/3 -> Discrete 2nd-Order Filter10/1
  Demux2/2 -> Discrete 2nd-Order Filter9/1
  Demux2/1 -> Discrete 2nd-Order Filter8/1
  Discrete 2nd-Order Filter7/1 -> "Vdc "/1
  Vdc/1 -> Discrete 2nd-Order Filter7/1
  Mux1/1 -> "Iabc_grid_conv "/1
  Iabc_grid_conv/1 -> Demux1/1
  Discrete 2nd-Order Filter4/1 -> Mux1/3
  Discrete 2nd-Order Filter6/1 -> Mux1/2
  Discrete 2nd-Order Filter5/1 -> Mux1/1
  Demux1/3 -> Discrete 2nd-Order Filter4/1
  Demux1/2 -> Discrete 2nd-Order Filter6/1
  Demux1/1 -> Discrete 2nd-Order Filter5/1
  Mux/1 -> "Vabc_B1 "/1
  Vabc_B1/1 -> Demux/1
  Discrete 2nd-Order Filter3/1 -> Mux/3
  Discrete 2nd-Order Filter2/1 -> Mux/2
  Discrete 2nd-Order Filter1/1 -> Mux/1
  Demux/3 -> Discrete 2nd-Order Filter3/1
  Demux/2 -> Discrete 2nd-Order Filter2/1
  Demux/1 -> Discrete 2nd-Order Filter1/1

== system GFL_inverter/PMSG Wind Turbine/Control/Rotor-side Controls/dq to ABC conversion  ==
  dq : Inport
  Teta : Inport  Port=2
  Fcn : Fcn  Expr=sin(u)
  Fcn1 : Fcn  Expr=cos(u)
  Mux : Mux  Inputs=[1 1 2]
  Mux1 : Mux  Inputs=3
  a : Fcn  Expr=u(1)*u(3)-u(2)*u(4)
  b : Fcn  Expr=(u(1)*(-0.5)+u(2)*(0.8660254))*u(3)-(u(2)*(-0.5)-u(1)*(0.8660254))*u(4)
  c : Fcn  Expr=(u(1)*(-0.5)-u(2)*(0.8660254))*u(3)-(u(2)*(-0.5)+u(1)*(0.8660254))*u(4)
  ABC : Outport
  wires:
  Fcn/1 -> Mux/2
  Fcn1/1 -> Mux/1
  Teta/1 -> Fcn1/1, Fcn/1
  Mux/1 -> a/1, b/1, c/1
  dq/1 -> Mux/3
  b/1 -> Mux1/2
  a/1 -> Mux1/1
  Mux1/1 -> ABC/1
  c/1 -> Mux1/3
